simulink library "tqd"  (R2021b)
settings: Solver=VariableStepAuto  StartTime=0.0  StopTime=10.0  RelTol=1e-3
undefined symbols (not defined in the file or in its folder): ATQD_AccelLimitInRange_X_rpm, ATQD_AccelLimitInRange_Y_Nm, ATQD_AccelLimitOvrKi_X_Nm, ATQD_AccelLimitOvrKp_X_Nm, ATQD_BOSMapD_X_rpm, ATQD_BOSMapD_Y_pct, ATQD_BOSMapR_X_rpm, ATQD_BOSMapR_Y_pct, ATQD_HVBCurrSmooth_X_A, ATQD_LHMTqMapDLC_X_rpm, ATQD_LHMTqMapDLC_Y_pct, ATQD_LHMTqMapRLC_X_rpm, ATQD_LHMTqMapRLC_Y_pct, ATQD_NormalMapDLC_X_rpm, ATQD_NormalMapDLC_Y_pct, ATQD_NormalTqDecSR_X_rpm, ATQD_NormalTqDecSR_Y_Nm, ATQD_NormalTqIncSR_X_rpm, ATQD_NormalTqIncSR_Y_Nm, ATQD_OPDMapRLC_X_rpm, ATQD_OPDMapRLC_Y_pct, ATQD_RollRegTorReq_X_rpm, ATQD_RollRegTorReq_Y_enum, ATQD_VehSpdLimitInRange_X_rpm, ATQD_VehSpdLimitInRange_Y_Nm, ATQD_VehSpdLimitOvrKi_X_Nm, ATQD_VehSpdLimitOvrKp_X_Nm, EIGHT_INT, ENUM_BRAKEPEDAL_PRESSED, ENUM_BRAKEPEDAL_RELEASED, ENUM_COMBOKEY_DOWN, ENUM_COMBOKEY_M1, ENUM_COMBOKEY_M2, ENUM_COMBOKEY_NONE, ENUM_COMBOKEY_RKNEE, ENUM_COMBOKEY_STOPLV, ENUM_COMBOKEY_UP, ENUM_CP2VKNEEREQ_REQUEST, ENUM_CP2VNLVREQ_LEVEL1, ENUM_CP2VNLVREQ_LEVEL2, ENUM_CP2VNLVREQ_LOWER, ENUM_CP2VNLVREQ_STOPLV, ENUM_CP2VNLVREQ_UPPER, ENUM_CREEPIND_DISABLE, ENUM_CREEPIND_READY, ENUM_CREEPIND_RUNNING, ENUM_CREEPIND_WARNING, ENUM_DRIVELINERELEASE_RELEASE, ENUM_EBSTORQUERWQ_LIMIT, ENUM_EBSTORQUERWQ_TORQUE, ENUM_ECPVCUDRM_CONFORT, ENUM_ECPVCUDRM_ECO, ENUM_ECPVCUDRM_NORMAL, ENUM_ECPVCUDRM_NOTAVAILABLE, ENUM_EMTqModeDrvBrk_Accel, ENUM_EMTqModeDrvBrk_Brake, ENUM_EMTqModeDrvBrk_Coast, ENUM_ETC2ACTDRIVEDIR_BACKWARD, ENUM_ETC2ACTDRIVEDIR_FORWARD, ENUM_ETC2ACTDRIVEDIR_STILL ... (+341)
libraries: simulink x109, hcu_lib x67
(part 9 of 13)

== system tqd/TQD/Input_Convert/Input Signal Convert/Big Mike Combo V2 /Combo Key Detection/Function3 ==
  note: Manufacture Mode:
      | 11 = VINP_SWC2RRightSta_flg
      | 12 = VINP_SWC2RLeftSta_flg
      | 11 = VINP_SWC2RRightSta_flg
      | 12 = VINP_SWC2RLeftSta_flg
      | 11 = VINP_SWC2RRightSta_flg
      | 12 = VINP_SWC2RLeftSta_flg
      | 7 = VINP_SWC2LScrollPressSta_flg
      | 8 = VINP_SWC2LADASSta_flg
  task_time_s : Inport
  VTQD_ComboKeyEn_flg : Inport  Port=2
  VTQD_ComboKeyReset_flg : Inport  Port=3
  VTQD_ComboKey_enum : Inport  Port=4
  VTQD_ComboKeyEnter_flg : Inport  Port=5
  VTQD_ComboKeyOff_flg : Inport  Port=6
  AND : Logic  Inputs=9  AllPortsSameDT=off  OutDataTypeStr=boolean
  AND1 : Logic  AllPortsSameDT=off  OutDataTypeStr=boolean
  Constant : Constant  Value=ENUM_COMBOKEY_NONE
  Constant1 : Constant  Value=ENUM_COMBOKEY_NONE
  Constant2 : Constant  Value=FALSE
  Constant3 : Constant  Value=KTQD_ComboKeyDelay_s
  Delay : Delay  DelayLength=1  InitialCondition=uint8(0)
      settings: AttributesFormatString=%<InitialCondition>
  Delay1 : Delay  DelayLength=1  InitialCondition=uint8(0)
      settings: AttributesFormatString=%<InitialCondition>
  DelayEnable : hcu_lib/Basic_Blocks/DelayEnable
  Equal : RelationalOperator  Operator=~=  OutDataTypeStr=boolean  RndMeth=Simplest
  Key1 : Subsystem
      settings: RTWSystemCode=Nonreusable function
  Key2 : Subsystem
      settings: RTWSystemCode=Nonreusable function
  Key3 : Subsystem
      settings: RTWSystemCode=Nonreusable function
  Key4 : Subsystem
      settings: RTWSystemCode=Nonreusable function
  Key5 : Subsystem
      settings: RTWSystemCode=Nonreusable function
  Key6 : Subsystem
      settings: RTWSystemCode=Nonreusable function
  Key7 : Subsystem
      settings: RTWSystemCode=Nonreusable function
  Key8 : Subsystem
      settings: RTWSystemCode=Nonreusable function
  NOT : Logic  Operator=NOT  AllPortsSameDT=off  OutDataTypeStr=boolean
  Switch : Switch  Criteria=u2 ~= 0
      settings: AttributesFormatString=%<Criteria>
  Switch1 : Switch  Criteria=u2 ~= 0
      settings: AttributesFormatString=%<Criteria>
  Switch2 : Switch  Criteria=u2 ~= 0
      settings: AttributesFormatString=%<Criteria>
  VTQD_Function3Off_flg : Outport
  wires:
  [VTQD_Function3Off_flg] -> VTQD_Function3Off_flg/1
  Switch/1 -> [VTQD_Function3CMD_enum]  "VTQD_Function3CMD_enum"
  [task_time_s] -> DelayEnable/3
  Constant/1 -> Switch/3
  DelayEnable/1 -> Switch/2
  [VTQD_ComboKeyEn_flg] -> DelayEnable/1
  Constant3/1 -> DelayEnable/2
  [VTQD_ComboKey_enum] -> Switch/1
  [VTQD_Function3CMD_enum] -> Key1/1(VTQD_ComboKeyCMD_enum)
  [VTQD_ComboKeyEn_flg] -> Key1/2(VTQD_ComboKeyEn_flg)
  [VTQD_ComboKeyReset_flg] -> Key1/3(VTQD_ComboKeyReset_flg)
  [VTQD_Function3CMD_enum] -> Key2/1(VTQD_ComboKeyCMD_enum)
  [VTQD_ComboKeyEn_flg] -> Key2/2(VTQD_ComboKeyEn_flg)
  [VTQD_ComboKeyReset_flg] -> Key2/3(VTQD_ComboKeyReset_flg)
  [VTQD_ComboKey1_enum] -> Key2/4(VTQD_ComboKey1_enum)
  Key1/1(VTQD_ComboKey1_enum) -> [VTQD_ComboKey1_enum]
  Key1/2(VTQD_Key1Pass_flg) -> [VTQD_Key1Pass_flg]
  [VTQD_Function3CMD_enum] -> Key3/1(VTQD_ComboKeyCMD_enum)
  [VTQD_ComboKeyEn_flg] -> Key3/2(VTQD_ComboKeyEn_flg)
  [VTQD_ComboKeyReset_flg] -> Key3/3(VTQD_ComboKeyReset_flg)
  [VTQD_ComboKey2_enum] -> Key3/4(VTQD_ComboKey2_enum)
  [VTQD_Function3CMD_enum] -> Key4/1(VTQD_ComboKeyCMD_enum)
  [VTQD_ComboKeyEn_flg] -> Key4/2(VTQD_ComboKeyEn_flg)
  [VTQD_ComboKeyReset_flg] -> Key4/3(VTQD_ComboKeyReset_flg)
  Key2/1(VTQD_ComboKey2_enum) -> [VTQD_ComboKey2_enum]
  Key2/2(VTQD_Key2Pass_flg) -> [VTQD_Key2Pass_flg]
  [VTQD_ComboKey3_enum] -> Key4/4(VTQD_ComboKey3_enum)
  Key3/1(VTQD_ComboKey3_enum) -> [VTQD_ComboKey3_enum]
  Key3/2(VTQD_Key3Pass_flg) -> [VTQD_Key3Pass_flg]
  Key4/1(VTQD_ComboKey4_enum) -> [VTQD_ComboKey4_enum]
  Key4/2(VTQD_Key4Pass_flg) -> [VTQD_Key4Pass_flg]
  [VTQD_ComboKeyReset_flg] -> Key5/3(VTQD_ComboKeyReset_flg)
  [VTQD_ComboKeyEn_flg] -> Key5/2(VTQD_ComboKeyEn_flg)
  [VTQD_Function3CMD_enum] -> Key5/1(VTQD_ComboKeyCMD_enum)
  [VTQD_ComboKey4_enum] -> Key5/4(VTQD_ComboKey4_enum)
  Key5/2(VTQD_Key5Pass_flg) -> [VTQD_Key5Pass_flg]
  Key5/1(VTQD_ComboKey5_enum) -> [VTQD_ComboKey5_enum]
  Key7/2(VTQD_Key7Pass_flg) -> [VTQD_Key7Pass_flg]
  Key8/1(VTQD_ComboKey8_enum) -> [VTQD_ComboKey8_enum]
  Key8/2(VTQD_Key8Pass_flg) -> [VTQD_Key8Pass_flg]
  [VTQD_Function3CMD_enum] -> Key6/1(VTQD_ComboKeyCMD_enum)
  [VTQD_ComboKeyEn_flg] -> Key6/2(VTQD_ComboKeyEn_flg)
  [VTQD_ComboKeyReset_flg] -> Key6/3(VTQD_ComboKeyReset_flg)
  [VTQD_ComboKey5_enum] -> Key6/4(VTQD_ComboKey5_enum)
  [VTQD_Function3CMD_enum] -> Key7/1(VTQD_ComboKeyCMD_enum)
  [VTQD_ComboKeyEn_flg] -> Key7/2(VTQD_ComboKeyEn_flg)
  [VTQD_ComboKeyReset_flg] -> Key7/3(VTQD_ComboKeyReset_flg)
  [VTQD_ComboKey6_enum] -> Key7/4(VTQD_ComboKey6_enum)
  [VTQD_Function3CMD_enum] -> Key8/1(VTQD_ComboKeyCMD_enum)
  [VTQD_ComboKeyEn_flg] -> Key8/2(VTQD_ComboKeyEn_flg)
  [VTQD_ComboKeyReset_flg] -> Key8/3(VTQD_ComboKeyReset_flg)
  [VTQD_ComboKey7_enum] -> Key8/4(VTQD_ComboKey7_enum)
  Constant1/1 -> Equal/2
  Equal/1 -> AND/1
  [VTQD_Key1Pass_flg] -> AND/2
  [VTQD_Key8Pass_flg] -> AND/9
  [VTQD_Key7Pass_flg] -> AND/8
  [VTQD_Key6Pass_flg] -> AND/7
  [VTQD_Key5Pass_flg] -> AND/6
  [VTQD_Key4Pass_flg] -> AND/5
  [VTQD_Key3Pass_flg] -> AND/4
  [VTQD_Key2Pass_flg] -> AND/3
  AND/1 -> Switch1/1  "VTQD_Function3OffPass_flg"
  Switch1/1 -> Switch2/3
  [VTQD_ComboKeyOff_flg] -> Switch2/2
  Constant2/1 -> Switch2/1
  Switch2/1 -> Delay/1, [VTQD_Function3Off_flg]  "VTQD_Function3Off_flg"
  Delay/1 -> Switch1/3
  task_time_s/1 -> [task_time_s]
  VTQD_ComboKeyEn_flg/1 -> [VTQD_ComboKeyEn_flg]
  VTQD_ComboKeyReset_flg/1 -> [VTQD_ComboKeyReset_flg]
  VTQD_ComboKey_enum/1 -> [VTQD_ComboKey_enum]
  VTQD_ComboKeyEnter_flg/1 -> [VTQD_ComboKeyEnter_flg]
  VTQD_ComboKeyOff_flg/1 -> [VTQD_ComboKeyOff_flg]
  Key6/1(VTQD_ComboKey6_enum) -> [VTQD_ComboKey6_enum]
  Key6/2(VTQD_Key6Pass_flg) -> [VTQD_Key6Pass_flg]
  Key7/1(VTQD_ComboKey7_enum) -> [VTQD_ComboKey7_enum]
  [VTQD_ComboKey8_enum] -> Equal/1
  NOT/1 -> AND1/2
  Delay1/1 -> NOT/1
  [VTQD_ComboKeyEnter_flg] -> AND1/1
  AND1/1 -> Switch1/2
  [VTQD_Function3Off_flg] -> Delay1/1

== system tqd/TQD/Input_Convert/Input Signal Convert/Big Mike Combo V2 /Combo Key Detection/Function4  ==
  note: Exhibition Mode:
      | 7 = VINP_SWC2LScrollPressSta_flg
      | 7 = VINP_SWC2LScrollPressSta_flg
      | 8 = VINP_SWC2LADASSta_flg
      | 8 = VINP_SWC2LADASSta_flg
      | 8 = VINP_SWC2LADASSta_flg
      | 7 = VINP_SWC2LScrollPressSta_flg
      | 8 = VINP_SWC2LADASSta_flg
      | 7 = VINP_SWC2LScrollPressSta_flg
  task_time_s : Inport
  VTQD_ComboKeyEn_flg : Inport  Port=2
  VTQD_ComboKeyReset_flg : Inport  Port=3
  VTQD_ComboKey_enum : Inport  Port=4
  VTQD_ComboKeyEnter_flg : Inport  Port=5
  VTQD_ComboKeyOff_flg : Inport  Port=6
  AND : Logic  Inputs=9  AllPortsSameDT=off  OutDataTypeStr=boolean
  AND1 : Logic  AllPortsSameDT=off  OutDataTypeStr=boolean
  Constant : Constant  Value=ENUM_COMBOKEY_NONE
  Constant1 : Constant  Value=ENUM_COMBOKEY_NONE
  Constant2 : Constant  Value=FALSE
  Constant3 : Constant  Value=KTQD_ComboKeyDelay_s
  Delay : Delay  DelayLength=1  InitialCondition=boolean(0)
      settings: AttributesFormatString=%<InitialCondition>
  Delay1 : Delay  DelayLength=1  InitialCondition=boolean(0)
      settings: AttributesFormatString=%<InitialCondition>
  DelayEnable : hcu_lib/Basic_Blocks/DelayEnable
  Equal : RelationalOperator  Operator=~=  OutDataTypeStr=boolean  RndMeth=Simplest
  Key1 : Subsystem
      settings: RTWSystemCode=Nonreusable function
  Key2 : Subsystem
      settings: RTWSystemCode=Nonreusable function
  Key3 : Subsystem
      settings: RTWSystemCode=Nonreusable function
  Key4 : Subsystem
      settings: RTWSystemCode=Nonreusable function
  Key5 : Subsystem
      settings: RTWSystemCode=Nonreusable function
  Key6 : Subsystem
      settings: RTWSystemCode=Nonreusable function
  Key7 : Subsystem
      settings: RTWSystemCode=Nonreusable function
  Key8 : Subsystem
      settings: RTWSystemCode=Nonreusable function
  NOT : Logic  Operator=NOT  AllPortsSameDT=off  OutDataTypeStr=boolean
  Switch : Switch  Criteria=u2 ~= 0
      settings: AttributesFormatString=%<Criteria>
  Switch1 : Switch  Criteria=u2 ~= 0
      settings: AttributesFormatString=%<Criteria>
  Switch2 : Switch  Criteria=u2 ~= 0
      settings: AttributesFormatString=%<Criteria>
  VTQD_Function4Off_flg : Outport
  wires:
  [VTQD_ComboKey8_enum] -> Equal/1
  Key7/1(VTQD_ComboKey7_enum) -> [VTQD_ComboKey7_enum]
  Key6/2(VTQD_Key6Pass_flg) -> [VTQD_Key6Pass_flg]
  Key6/1(VTQD_ComboKey6_enum) -> [VTQD_ComboKey6_enum]
  VTQD_ComboKeyOff_flg/1 -> [VTQD_ComboKeyOff_flg]
  VTQD_ComboKeyEnter_flg/1 -> [VTQD_ComboKeyEnter_flg]
  VTQD_ComboKey_enum/1 -> [VTQD_ComboKey_enum]
  VTQD_ComboKeyReset_flg/1 -> [VTQD_ComboKeyReset_flg]
  VTQD_ComboKeyEn_flg/1 -> [VTQD_ComboKeyEn_flg]
  task_time_s/1 -> [task_time_s]
  Delay/1 -> Switch1/3
  Switch2/1 -> [VTQD_Function4Off_flg], Delay/1  "VTQD_Function4Off_flg"
  Constant2/1 -> Switch2/1
  [VTQD_ComboKeyOff_flg] -> Switch2/2
  Switch1/1 -> Switch2/3
  AND/1 -> Switch1/1  "VTQD_Function4OffPass_flg"
  [VTQD_Key2Pass_flg] -> AND/3
  [VTQD_Key3Pass_flg] -> AND/4
  [VTQD_Key4Pass_flg] -> AND/5
  [VTQD_Key5Pass_flg] -> AND/6
  [VTQD_Key6Pass_flg] -> AND/7
  [VTQD_Key7Pass_flg] -> AND/8
  [VTQD_Key8Pass_flg] -> AND/9
  [VTQD_Key1Pass_flg] -> AND/2
  Equal/1 -> AND/1
  Constant1/1 -> Equal/2
  [VTQD_ComboKey7_enum] -> Key8/4(VTQD_ComboKey7_enum)
  [VTQD_ComboKeyReset_flg] -> Key8/3(VTQD_ComboKeyReset_flg)
  [VTQD_ComboKeyEn_flg] -> Key8/2(VTQD_ComboKeyEn_flg)
  [VTQD_Function4CMD_enum] -> Key8/1(VTQD_ComboKeyCMD_enum)
  [VTQD_ComboKey6_enum] -> Key7/4(VTQD_ComboKey6_enum)
  [VTQD_ComboKeyReset_flg] -> Key7/3(VTQD_ComboKeyReset_flg)
  [VTQD_ComboKeyEn_flg] -> Key7/2(VTQD_ComboKeyEn_flg)
  [VTQD_Function4CMD_enum] -> Key7/1(VTQD_ComboKeyCMD_enum)
  [VTQD_ComboKey5_enum] -> Key6/4(VTQD_ComboKey5_enum)
  [VTQD_ComboKeyReset_flg] -> Key6/3(VTQD_ComboKeyReset_flg)
  [VTQD_ComboKeyEn_flg] -> Key6/2(VTQD_ComboKeyEn_flg)
  [VTQD_Function4CMD_enum] -> Key6/1(VTQD_ComboKeyCMD_enum)
  Key8/2(VTQD_Key8Pass_flg) -> [VTQD_Key8Pass_flg]
  Key8/1(VTQD_ComboKey8_enum) -> [VTQD_ComboKey8_enum]
  Key7/2(VTQD_Key7Pass_flg) -> [VTQD_Key7Pass_flg]
  Key5/1(VTQD_ComboKey5_enum) -> [VTQD_ComboKey5_enum]
  Key5/2(VTQD_Key5Pass_flg) -> [VTQD_Key5Pass_flg]
  [VTQD_ComboKey4_enum] -> Key5/4(VTQD_ComboKey4_enum)
  [VTQD_Function4CMD_enum] -> Key5/1(VTQD_ComboKeyCMD_enum)
  [VTQD_ComboKeyEn_flg] -> Key5/2(VTQD_ComboKeyEn_flg)
  [VTQD_ComboKeyReset_flg] -> Key5/3(VTQD_ComboKeyReset_flg)
  Key4/2(VTQD_Key4Pass_flg) -> [VTQD_Key4Pass_flg]
  Key4/1(VTQD_ComboKey4_enum) -> [VTQD_ComboKey4_enum]
  Key3/2(VTQD_Key3Pass_flg) -> [VTQD_Key3Pass_flg]
  Key3/1(VTQD_ComboKey3_enum) -> [VTQD_ComboKey3_enum]
  [VTQD_ComboKey3_enum] -> Key4/4(VTQD_ComboKey3_enum)
  Key2/2(VTQD_Key2Pass_flg) -> [VTQD_Key2Pass_flg]
  Key2/1(VTQD_ComboKey2_enum) -> [VTQD_ComboKey2_enum]
  [VTQD_ComboKeyReset_flg] -> Key4/3(VTQD_ComboKeyReset_flg)
  [VTQD_ComboKeyEn_flg] -> Key4/2(VTQD_ComboKeyEn_flg)
  [VTQD_Function4CMD_enum] -> Key4/1(VTQD_ComboKeyCMD_enum)
  [VTQD_ComboKey2_enum] -> Key3/4(VTQD_ComboKey2_enum)
  [VTQD_ComboKeyReset_flg] -> Key3/3(VTQD_ComboKeyReset_flg)
  [VTQD_ComboKeyEn_flg] -> Key3/2(VTQD_ComboKeyEn_flg)
  [VTQD_Function4CMD_enum] -> Key3/1(VTQD_ComboKeyCMD_enum)
  Key1/2(VTQD_Key1Pass_flg) -> [VTQD_Key1Pass_flg]
  Key1/1(VTQD_ComboKey1_enum) -> [VTQD_ComboKey1_enum]
  [VTQD_ComboKey1_enum] -> Key2/4(VTQD_ComboKey1_enum)
  [VTQD_ComboKeyReset_flg] -> Key2/3(VTQD_ComboKeyReset_flg)
  [VTQD_ComboKeyEn_flg] -> Key2/2(VTQD_ComboKeyEn_flg)
  [VTQD_Function4CMD_enum] -> Key2/1(VTQD_ComboKeyCMD_enum)
  [VTQD_ComboKeyReset_flg] -> Key1/3(VTQD_ComboKeyReset_flg)
  [VTQD_ComboKeyEn_flg] -> Key1/2(VTQD_ComboKeyEn_flg)
  [VTQD_Function4CMD_enum] -> Key1/1(VTQD_ComboKeyCMD_enum)
  [VTQD_ComboKey_enum] -> Switch/1
  Constant3/1 -> DelayEnable/2
  [VTQD_ComboKeyEn_flg] -> DelayEnable/1
  DelayEnable/1 -> Switch/2
  Constant/1 -> Switch/3
  [task_time_s] -> DelayEnable/3
  Switch/1 -> [VTQD_Function4CMD_enum]  "VTQD_Function4CMD_enum"
  [VTQD_Function4Off_flg] -> VTQD_Function4Off_flg/1
  NOT/1 -> AND1/2
  Delay1/1 -> NOT/1
  [VTQD_Function4Off_flg] -> Delay1/1
  [VTQD_ComboKeyEnter_flg] -> AND1/1
  AND1/1 -> Switch1/2

== system tqd/TQD/Input_Convert/Input Signal Convert/Big Mike Combo V2 /Combo Key Detection/Function5 ==
  note: Exhibition Mode:
      | 1 = VINP_SWC2RegenDown_flg
      | 2 = VINP_SWC2RegenUp_flg
      | 3 = VINP_SWC2LScrollUpSta_flg
      | 4 = VINP_SWC2LScrollDownSta_flg
      | 5 = VINP_SWC2RScrollUpSta_flg
      | 6 = VINP_SWC2RScrollDownSta_flg
      | 7 = VINP_SWC2LScrollPressSta_flg
      | 8 = VINP_SWC2LADASSta_flg
  task_time_s : Inport
  VTQD_ComboKeyEn_flg : Inport  Port=2
  VTQD_ComboKeyReset_flg : Inport  Port=3
  VTQD_ComboKey_enum : Inport  Port=4
  VTQD_ComboKeyEnter_flg : Inport  Port=5
  VTQD_ComboKeyOff_flg : Inport  Port=6
  AND : Logic  Inputs=9  AllPortsSameDT=off  OutDataTypeStr=boolean
  AND1 : Logic  AllPortsSameDT=off  OutDataTypeStr=boolean
  Constant : Constant  Value=ENUM_COMBOKEY_NONE
  Constant1 : Constant  Value=ENUM_COMBOKEY_NONE
  Constant2 : Constant  Value=FALSE
  Constant3 : Constant  Value=KTQD_ComboKeyDelay_s
  Delay : Delay  DelayLength=1  InitialCondition=uint8(0)
      settings: AttributesFormatString=%<InitialCondition>
  Delay1 : Delay  DelayLength=1  InitialCondition=boolean(0)
      settings: AttributesFormatString=%<InitialCondition>
  DelayEnable : hcu_lib/Basic_Blocks/DelayEnable
  Equal : RelationalOperator  Operator=~=  OutDataTypeStr=boolean  RndMeth=Simplest
  Key1 : Subsystem
      settings: RTWSystemCode=Nonreusable function
  Key2 : Subsystem
      settings: RTWSystemCode=Nonreusable function
  Key3 : Subsystem
      settings: RTWSystemCode=Nonreusable function
  Key4 : Subsystem
      settings: RTWSystemCode=Nonreusable function
  Key5 : Subsystem
      settings: RTWSystemCode=Nonreusable function
  Key6 : Subsystem
      settings: RTWSystemCode=Nonreusable function
  Key7 : Subsystem
      settings: RTWSystemCode=Nonreusable function
  Key8 : Subsystem
      settings: RTWSystemCode=Nonreusable function
  NOT : Logic  Operator=NOT  AllPortsSameDT=off  OutDataTypeStr=boolean
  Switch : Switch  Criteria=u2 ~= 0
      settings: AttributesFormatString=%<Criteria>
  Switch1 : Switch  Criteria=u2 ~= 0
      settings: AttributesFormatString=%<Criteria>
  Switch2 : Switch  Criteria=u2 ~= 0
      settings: AttributesFormatString=%<Criteria>
  VTQD_Function5Off_flg : Outport
  wires:
  [VTQD_Function5Off_flg] -> VTQD_Function5Off_flg/1
  Switch/1 -> [VTQD_Function5CMD_enum]  "VTQD_Function5CMD_enum"
  [task_time_s] -> DelayEnable/3
  Constant/1 -> Switch/3
  DelayEnable/1 -> Switch/2
  [VTQD_ComboKeyEn_flg] -> DelayEnable/1
  Constant3/1 -> DelayEnable/2
  [VTQD_ComboKey_enum] -> Switch/1
  [VTQD_Function5CMD_enum] -> Key1/1(VTQD_ComboKeyCMD_enum)
  [VTQD_ComboKeyEn_flg] -> Key1/2(VTQD_ComboKeyEn_flg)
  [VTQD_ComboKeyReset_flg] -> Key1/3(VTQD_ComboKeyReset_flg)
  [VTQD_Function5CMD_enum] -> Key2/1(VTQD_ComboKeyCMD_enum)
  [VTQD_ComboKeyEn_flg] -> Key2/2(VTQD_ComboKeyEn_flg)
  [VTQD_ComboKeyReset_flg] -> Key2/3(VTQD_ComboKeyReset_flg)
  [VTQD_ComboKey1_enum] -> Key2/4(VTQD_ComboKey1_enum)
  Key1/1(VTQD_ComboKey1_enum) -> [VTQD_ComboKey1_enum]
  Key1/2(VTQD_Key1Pass_flg) -> [VTQD_Key1Pass_flg]
  [VTQD_Function5CMD_enum] -> Key3/1(VTQD_ComboKeyCMD_enum)
  [VTQD_ComboKeyEn_flg] -> Key3/2(VTQD_ComboKeyEn_flg)
  [VTQD_ComboKeyReset_flg] -> Key3/3(VTQD_ComboKeyReset_flg)
  [VTQD_ComboKey2_enum] -> Key3/4(VTQD_ComboKey2_enum)
  [VTQD_Function5CMD_enum] -> Key4/1(VTQD_ComboKeyCMD_enum)
  [VTQD_ComboKeyEn_flg] -> Key4/2(VTQD_ComboKeyEn_flg)
  [VTQD_ComboKeyReset_flg] -> Key4/3(VTQD_ComboKeyReset_flg)
  Key2/1(VTQD_ComboKey2_enum) -> [VTQD_ComboKey2_enum]
  Key2/2(VTQD_Key2Pass_flg) -> [VTQD_Key2Pass_flg]
  [VTQD_ComboKey3_enum] -> Key4/4(VTQD_ComboKey3_enum)
  Key3/1(VTQD_ComboKey3_enum) -> [VTQD_ComboKey3_enum]
  Key3/2(VTQD_Key3Pass_flg) -> [VTQD_Key3Pass_flg]
  Key4/1(VTQD_ComboKey4_enum) -> [VTQD_ComboKey4_enum]
  Key4/2(VTQD_Key4Pass_flg) -> [VTQD_Key4Pass_flg]
  [VTQD_ComboKeyReset_flg] -> Key5/3(VTQD_ComboKeyReset_flg)
  [VTQD_ComboKeyEn_flg] -> Key5/2(VTQD_ComboKeyEn_flg)
  [VTQD_Function5CMD_enum] -> Key5/1(VTQD_ComboKeyCMD_enum)
  [VTQD_ComboKey4_enum] -> Key5/4(VTQD_ComboKey4_enum)
  Key5/2(VTQD_Key5Pass_flg) -> [VTQD_Key5Pass_flg]
  Key5/1(VTQD_ComboKey5_enum) -> [VTQD_ComboKey5_enum]
  Key7/2(VTQD_Key7Pass_flg) -> [VTQD_Key7Pass_flg]
  Key8/1(VTQD_ComboKey8_enum) -> [VTQD_ComboKey8_enum]
  Key8/2(VTQD_Key8Pass_flg) -> [VTQD_Key8Pass_flg]
  [VTQD_Function5CMD_enum] -> Key6/1(VTQD_ComboKeyCMD_enum)
  [VTQD_ComboKeyEn_flg] -> Key6/2(VTQD_ComboKeyEn_flg)
  [VTQD_ComboKeyReset_flg] -> Key6/3(VTQD_ComboKeyReset_flg)
  [VTQD_ComboKey5_enum] -> Key6/4(VTQD_ComboKey5_enum)
  [VTQD_Function5CMD_enum] -> Key7/1(VTQD_ComboKeyCMD_enum)
  [VTQD_ComboKeyEn_flg] -> Key7/2(VTQD_ComboKeyEn_flg)
  [VTQD_ComboKeyReset_flg] -> Key7/3(VTQD_ComboKeyReset_flg)
  [VTQD_ComboKey6_enum] -> Key7/4(VTQD_ComboKey6_enum)
  [VTQD_Function5CMD_enum] -> Key8/1(VTQD_ComboKeyCMD_enum)
  [VTQD_ComboKeyEn_flg] -> Key8/2(VTQD_ComboKeyEn_flg)
  [VTQD_ComboKeyReset_flg] -> Key8/3(VTQD_ComboKeyReset_flg)
  [VTQD_ComboKey7_enum] -> Key8/4(VTQD_ComboKey7_enum)
  Constant1/1 -> Equal/2
  Equal/1 -> AND/1
  [VTQD_Key1Pass_flg] -> AND/2
  [VTQD_Key8Pass_flg] -> AND/9
  [VTQD_Key7Pass_flg] -> AND/8
  [VTQD_Key6Pass_flg] -> AND/7
  [VTQD_Key5Pass_flg] -> AND/6
  [VTQD_Key4Pass_flg] -> AND/5
  [VTQD_Key3Pass_flg] -> AND/4
  [VTQD_Key2Pass_flg] -> AND/3
  AND/1 -> Switch1/1  "VTQD_Function5OffPass_flg"
  Switch1/1 -> Switch2/3
  [VTQD_ComboKeyOff_flg] -> Switch2/2
  Constant2/1 -> Switch2/1
  Switch2/1 -> [VTQD_Function5Off_flg], Delay/1  "VTQD_Function5Off_flg"
  Delay/1 -> Switch1/3
  task_time_s/1 -> [task_time_s]
  VTQD_ComboKeyEn_flg/1 -> [VTQD_ComboKeyEn_flg]
  VTQD_ComboKeyReset_flg/1 -> [VTQD_ComboKeyReset_flg]
  VTQD_ComboKey_enum/1 -> [VTQD_ComboKey_enum]
  VTQD_ComboKeyEnter_flg/1 -> [VTQD_ComboKeyEnter_flg]
  VTQD_ComboKeyOff_flg/1 -> [VTQD_ComboKeyOff_flg]
  Key6/1(VTQD_ComboKey6_enum) -> [VTQD_ComboKey6_enum]
  Key6/2(VTQD_Key6Pass_flg) -> [VTQD_Key6Pass_flg]
  Key7/1(VTQD_ComboKey7_enum) -> [VTQD_ComboKey7_enum]
  [VTQD_ComboKey8_enum] -> Equal/1
  NOT/1 -> AND1/2
  Delay1/1 -> NOT/1
  [VTQD_ComboKeyEnter_flg] -> AND1/1
  [VTQD_Function5Off_flg] -> Delay1/1
  AND1/1 -> Switch1/2

== system tqd/TQD/Input_Convert/Input Signal Convert/Big Mike Combo V2 /Signal Status Detection/DownShort ==
  Action Port : ActionPort
  Constant : Constant  Value=ENUM_COMBOKEY_DOWN  OutDataTypeStr=uint8
  DownShort : Outport
  wires:
  Constant/1 -> DownShort/1

== system tqd/TQD/Input_Convert/Input Signal Convert/Big Mike Combo V2 /Signal Status Detection/M1Short ==
  Action Port : ActionPort
  Constant : Constant  Value=ENUM_COMBOKEY_M1  OutDataTypeStr=uint8
  M1Short : Outport
  wires:
  Constant/1 -> M1Short/1

== system tqd/TQD/Input_Convert/Input Signal Convert/Big Mike Combo V2 /Signal Status Detection/M2Short ==
  Action Port : ActionPort
  Constant : Constant  Value=ENUM_COMBOKEY_M2  OutDataTypeStr=uint8
  M2Short : Outport
  wires:
  Constant/1 -> M2Short/1

== system tqd/TQD/Input_Convert/Input Signal Convert/Big Mike Combo V2 /Signal Status Detection/None ==
  Action Port : ActionPort
  Constant : Constant  Value=ENUM_COMBOKEY_NONE  OutDataTypeStr=uint8
  None : Outport
  wires:
  Constant/1 -> None/1

== system tqd/TQD/Input_Convert/Input Signal Convert/Big Mike Combo V2 /Signal Status Detection/RKneeShort ==
  Action Port : ActionPort
  Constant : Constant  Value=ENUM_COMBOKEY_RKNEE  OutDataTypeStr=uint8
  RKneeShort : Outport
  wires:
  Constant/1 -> RKneeShort/1

== system tqd/TQD/Input_Convert/Input Signal Convert/Big Mike Combo V2 /Signal Status Detection/StopLVShort ==
  Action Port : ActionPort
  Constant : Constant  Value=ENUM_COMBOKEY_STOPLV  OutDataTypeStr=uint8
  STOPLV : Outport
  wires:
  Constant/1 -> STOPLV/1

== system tqd/TQD/Input_Convert/Input Signal Convert/Big Mike Combo V2 /Signal Status Detection/Street Fight Switch Off ==
  task_time_s : Inport
  VTQD_SWCCANCELStaShort_flg : Inport  Port=2
  VTQD_ComboKeyPreEn_flg : Inport  Port=3
  SWCCANCELStaLong_flg : Inport  Port=4
  VTQD_FunctionOffSta_enum : Inport  Port=5
  AND : Logic  AllPortsSameDT=off  OutDataTypeStr=boolean
  AND2 : Logic  AllPortsSameDT=off  OutDataTypeStr=boolean
  Add : Sum
  Constant1 : Constant  Value=ZERO_INT
  Constant11 : Constant  Value=ONE_INT
  Constant2 : Constant  Value=ONE_INT
  Constant3 : Constant  Value=KTQD_CANCELUpCount_cnt
  Constant4 : Constant  Value=ZERO_INT
  Constant5 : Constant  Value=ZERO_INT
  Constant6 : Constant  Value=KTQD_ComboKeyOff_flg_ovrdflg
  Constant7 : Constant  Value=KTQD_CANCELCountDetTime_s
  Constant8 : Constant  Value=KTQD_ComboKeyOff_flg_ovrdval
  Delay : Delay  DelayLength=1  InitialCondition=uint8(0)
      settings: AttributesFormatString=%<InitialCondition>
  Delay1 : Delay  DelayLength=1  InitialCondition=boolean(0)
      settings: AttributesFormatString=%<InitialCondition>
  Delay2 : Delay  DelayLength=1  InitialCondition=boolean(0)
      settings: AttributesFormatString=%<InitialCondition>
  Delay3 : Delay  DelayLength=1  InitialCondition=uint8(0)
      settings: AttributesFormatString=%<InitialCondition>
  Equal : RelationalOperator  Operator===  OutDataTypeStr=boolean  RndMeth=Simplest
  Equal1 : RelationalOperator  Operator===  OutDataTypeStr=boolean  RndMeth=Simplest
  Equal2 : RelationalOperator  Operator=>  OutDataTypeStr=boolean  RndMeth=Simplest
  NOT : Logic  Operator=NOT  AllPortsSameDT=off  OutDataTypeStr=boolean
  NOT1 : Logic  Operator=NOT  AllPortsSameDT=off  OutDataTypeStr=boolean
  OR : Logic  Operator=OR  Inputs=3  AllPortsSameDT=off  OutDataTypeStr=boolean
  Relational Operator : RelationalOperator  OutDataTypeStr=boolean  RndMeth=Simplest
  SR_Latch : hcu_lib/Basic_Blocks/SR_Latch
  Switch : Switch  Criteria=u2 ~= 0
      settings: AttributesFormatString=%<Criteria>
  Switch1 : Switch  Criteria=u2 ~= 0
      settings: AttributesFormatString=%<Criteria>
  Switch2 : Switch  Criteria=u2 ~= 0
      settings: AttributesFormatString=%<Criteria>
  Timer : hcu_lib/Basic_Blocks/Timer
  VTQD_ComboKeyOff_flg : Outport
  wires:
  Constant1/1 -> Switch/3
  [VTQD_SWCCANCELStaShort_flg] -> Switch/2
  Constant11/1 -> Switch/1
  Switch/1 -> Add/1
  Add/1 -> Switch1/3
  Switch1/1 -> [VTQD_CANCELCount_cnt], Delay/1  "VTQD_CANCELCount_cnt"
  Delay/1 -> Add/2
  [VTQD_CANCELCount_cnt] -> Equal/1
  Constant2/1 -> Equal/2
  Equal/1 -> AND/1
  [VTQD_ComboKeyPreEn_flg] -> AND/2
  AND/1 -> SR_Latch/1
  SR_Latch/1 -> NOT/1, Timer/1
  NOT/1 -> Timer/2
  [task_time_s] -> Timer/3
  Constant7/1 -> Relational Operator/2, Timer/4
  Timer/1 -> Relational Operator/1  "VTQD_CANCELCountDetTime_s"
  Relational Operator/1 -> [VTQD_CANCELCountDetFinish_flg]  "VTQD_CANCELCountDetFinish_flg"
  [VTQD_CANCELCount_cnt] -> Equal1/1
  Constant3/1 -> Equal1/2
  [SWCCANCELStaLong_flg] -> AND2/2
  [VTQD_CANCELCountDetFinish_flg] -> Delay1/1
  Delay1/1 -> SR_Latch/2
  [VTQD_CANCELCountDetFinish_flg] -> Delay2/1
  Constant4/1 -> Switch1/1
  Equal1/1 -> AND2/1
  task_time_s/1 -> [task_time_s]
  VTQD_SWCCANCELStaShort_flg/1 -> [VTQD_SWCCANCELStaShort_flg]
  VTQD_ComboKeyPreEn_flg/1 -> [VTQD_ComboKeyPreEn_flg]
  SWCCANCELStaLong_flg/1 -> [SWCCANCELStaLong_flg]
  [VTQD_ComboKeyOff_flg] -> VTQD_ComboKeyOff_flg/1
  [VTQD_ComboKeyPreEn_flg] -> NOT1/1
  VTQD_FunctionOffSta_enum/1 -> [VTQD_FunctionOffSta_enum]
  Equal2/1 -> OR/1
  NOT1/1 -> OR/2
  Delay2/1 -> OR/3
  OR/1 -> [VTQD_CANCELCountReset_flg]  "VTQD_CANCELCountReset_flg"
  [VTQD_CANCELCountReset_flg] -> Switch1/2
  [VTQD_FunctionOffSta_enum] -> Delay3/1
  Delay3/1 -> Equal2/1
  Constant5/1 -> Equal2/2
  AND2/1 -> Switch2/3
  Constant6/1 -> Switch2/2
  Constant8/1 -> Switch2/1
  Switch2/1 -> [VTQD_ComboKeyOff_flg]  "VTQD_ComboKeyOff_flg"

== system tqd/TQD/Input_Convert/Input Signal Convert/Big Mike Combo V2 /Signal Status Detection/UpShort ==
  Action Port : ActionPort
  Constant : Constant  Value=ENUM_COMBOKEY_UP  OutDataTypeStr=uint8
  UpShort : Outport
  wires:
  Constant/1 -> UpShort/1

== system tqd/TQD/Input_Convert/Input Signal Convert/Big Mike Combo V2 /Combo Key Detection/Function1 Alcohol Lock/Key1 ==
  VTQD_ComboKeyCMD_enum : Inport
  VTQD_ComboKeyEn_flg : Inport  Port=2
  VTQD_ComboKeyReset_flg : Inport  Port=3
  AND : Logic  Inputs=3  AllPortsSameDT=off  OutDataTypeStr=boolean
  Constant1 : Constant  Value=KTQD_Function1Off1_enum
  Constant2 : Constant  Value=ENUM_COMBOKEY_NONE
  Constant4 : Constant  Value=ENUM_COMBOKEY_NONE
  Data Type Conversion : DataTypeConversion  OutDataTypeStr=uint8
  Delay : Delay  DelayLength=1  InitialCondition=uint8(0)
      settings: AttributesFormatString=%<InitialCondition>
  Delay1 : Delay  DelayLength=1  InitialCondition=uint8(0)
      settings: AttributesFormatString=%<InitialCondition>
  Detect Change : simulink/Logic and Bit Operations/Detect Change  vinit=boolean(0)  OutDataTypeStr=boolean
  Detect Increase : simulink/Logic and Bit Operations/Detect Increase  vinit=boolean(0)  OutDataTypeStr=boolean
  Equal : RelationalOperator  Operator===  OutDataTypeStr=boolean  RndMeth=Simplest
  Equal1 : RelationalOperator  Operator=~=  OutDataTypeStr=boolean  RndMeth=Simplest
  Equal2 : RelationalOperator  Operator===  OutDataTypeStr=boolean  RndMeth=Simplest
  If : If  NumInputs=2  IfExpression=u1 ~=0  ElseIfExpressions=u2 ~= 0
  Maintain : Subsystem  TreatAsAtomicUnit=on
  Merge : Merge  Inputs=3
  OR : Logic  Operator=OR  AllPortsSameDT=off  OutDataTypeStr=boolean
  Reset : Subsystem  TreatAsAtomicUnit=on
  Write : Subsystem  TreatAsAtomicUnit=on
  VTQD_ComboKey1_enum : Outport
  VTQD_Key1Pass_flg : Outport  Port=2
  wires:
  OR/1 -> [VTQD_ResetComboKey_flg]  "VTQD_ResetComboKey_flg"
  [VTQD_WriteComboCMD_flg] -> If/2
  [VTQD_ComboKeyCMD_enum] -> Equal1/1
  [VTQD_ComboKeyReset_flg] -> OR/2
  [VTQD_ComboKey1_enum] -> Delay/1
  Equal1/1 -> AND/2
  Constant2/1 -> Equal2/2
  Equal2/1 -> AND/3
  Reset/1(ResetToZero) -> Merge/1
  Merge/1 -> Data Type Conversion/1
  Delay/1 -> Equal2/1
  If/3 -> Maintain/Action
  Constant4/1 -> Equal1/2
  Maintain/1(KeepKey1) -> Merge/3
  Detect Change/1 -> AND/1
  [VTQD_ComboKeyEn_flg] -> Detect Increase/1
  [VTQD_ResetComboKey_flg] -> If/1
  [VTQD_ComboKeyCMD_enum] -> Detect Change/1
  [VTQD_ComboKeyCMD_enum] -> Write/1(Input)
  AND/1 -> [VTQD_WriteComboCMD_flg]  "VTQD_WriteComboCMD_flg"
  Detect Increase/1 -> OR/1
  If/1 -> Reset/Action
  Write/1(WriteCMD) -> Merge/2
  If/2 -> Write/Action
  [VTQD_ComboKey1_enum] -> Equal/1
  Constant1/1 -> Equal/2
  Equal/1 -> [VTQD_Function1Off1Pass_flg]  "VTQD_Function1Off1Pass_flg"
  VTQD_ComboKeyCMD_enum/1 -> [VTQD_ComboKeyCMD_enum]
  VTQD_ComboKeyReset_flg/1 -> [VTQD_ComboKeyReset_flg]
  VTQD_ComboKeyEn_flg/1 -> [VTQD_ComboKeyEn_flg]
  [VTQD_ComboKey1_enum] -> VTQD_ComboKey1_enum/1
  [VTQD_Function1Off1Pass_flg] -> VTQD_Key1Pass_flg/1
  [VTQD_ComboKey1_enum] -> Delay1/1
  Delay1/1 -> Maintain/1(Input)
  Data Type Conversion/1 -> [VTQD_ComboKey1_enum]  "VTQD_Function1Off1_enum"

== system tqd/TQD/Input_Convert/Input Signal Convert/Big Mike Combo V2 /Combo Key Detection/Function1 Alcohol Lock/Key2 ==
  VTQD_Function1CMD_enum : Inport
  VTQD_ComboKeyEn_flg : Inport  Port=2
  VTQD_ComboKeyReset_flg : Inport  Port=3
  VTQD_ComboKey1_enum : Inport  Port=4
  AND : Logic  Inputs=4  AllPortsSameDT=off  OutDataTypeStr=boolean
  Constant1 : Constant  Value=KTQD_Function1Off2_enum
  Constant2 : Constant  Value=ENUM_COMBOKEY_NONE
  Constant3 : Constant  Value=ENUM_COMBOKEY_NONE
  Constant4 : Constant  Value=ENUM_COMBOKEY_NONE  OutDataTypeStr=uint8
  Data Type Conversion : DataTypeConversion  OutDataTypeStr=uint8
  Delay : Delay  DelayLength=1  InitialCondition=uint8(0)
      settings: AttributesFormatString=%<InitialCondition>
  Delay1 : Delay  DelayLength=1  InitialCondition=uint8(0)
      settings: AttributesFormatString=%<InitialCondition>
  Delay2 : Delay  DelayLength=1  InitialCondition=uint8(0)
      settings: AttributesFormatString=%<InitialCondition>
  Detect Change : simulink/Logic and Bit Operations/Detect Change  vinit=boolean(0)  OutDataTypeStr=boolean
  Detect Increase : simulink/Logic and Bit Operations/Detect Increase  vinit=boolean(0)  OutDataTypeStr=boolean
  Equal : RelationalOperator  Operator===  OutDataTypeStr=boolean  RndMeth=Simplest
  Equal1 : RelationalOperator  Operator=~=  OutDataTypeStr=boolean  RndMeth=Simplest
  Equal2 : RelationalOperator  Operator=~=  OutDataTypeStr=boolean  RndMeth=Simplest
  Equal3 : RelationalOperator  Operator===  OutDataTypeStr=boolean  RndMeth=Simplest
  If : If  NumInputs=2  IfExpression=u1 ~=0  ElseIfExpressions=u2 ~= 0
  Maintain : Subsystem  TreatAsAtomicUnit=on
  Merge : Merge  Inputs=3
  OR : Logic  Operator=OR  AllPortsSameDT=off  OutDataTypeStr=boolean
  Reset : Subsystem  TreatAsAtomicUnit=on
  Write : Subsystem  TreatAsAtomicUnit=on
  VTQD_ComboKey2_enum : Outport
  VTQD_Key2Pass_flg : Outport  Port=2
  wires:
  [VTQD_Key2Pass_flg] -> VTQD_Key2Pass_flg/1
  [VTQD_ComboKey2_enum] -> VTQD_ComboKey2_enum/1
  VTQD_ComboKeyEn_flg/1 -> [VTQD_ComboKeyEn_flg]
  VTQD_ComboKeyReset_flg/1 -> [VTQD_ComboKeyReset_flg]
  VTQD_Function1CMD_enum/1 -> [VTQD_ComboKeyCMD_enum]
  Equal/1 -> [VTQD_Key2Pass_flg]  "VTQD_Function1Off2Pass_flg"
  Constant1/1 -> Equal/2
  [VTQD_ComboKey2_enum] -> Equal/1
  If/2 -> Write/Action
  Write/1(WriteCMD) -> Merge/2
  If/1 -> Reset/Action
  Detect Increase/1 -> OR/1
  AND/1 -> [VTQD_WriteComboCMD_flg]  "VTQD_WriteComboCMD_flg"
  [VTQD_ComboKeyCMD_enum] -> Write/1(Input)
  [VTQD_ComboKeyCMD_enum] -> Detect Change/1
  [VTQD_ResetComboKey_flg] -> If/1
  [VTQD_ComboKeyEn_flg] -> Detect Increase/1
  Detect Change/1 -> AND/1
  Maintain/1(KeepKey2) -> Merge/3
  Constant4/1 -> Equal1/2
  If/3 -> Maintain/Action
  Delay/1 -> Equal2/1
  Merge/1 -> Data Type Conversion/1
  Reset/1(ResetToZero) -> Merge/1
  Equal2/1 -> AND/3
  Constant2/1 -> Equal2/2
  Equal1/1 -> AND/2
  [VTQD_ComboKey1_enum] -> Delay/1
  [VTQD_ComboKeyReset_flg] -> OR/2
  [VTQD_ComboKeyCMD_enum] -> Equal1/1
  [VTQD_WriteComboCMD_flg] -> If/2
  OR/1 -> [VTQD_ResetComboKey_flg]  "VTQD_ResetComboKey_flg"
  VTQD_ComboKey1_enum/1 -> [VTQD_ComboKey1_enum]
  [VTQD_ComboKey2_enum] -> Delay1/1
  Constant3/1 -> Equal3/2
  Delay1/1 -> Equal3/1
  Equal3/1 -> AND/4
  Delay2/1 -> Maintain/1(Input)
  [VTQD_ComboKey2_enum] -> Delay2/1
  Data Type Conversion/1 -> [VTQD_ComboKey2_enum]  "VTQD_Function1Off2_enum"

== system tqd/TQD/Input_Convert/Input Signal Convert/Big Mike Combo V2 /Combo Key Detection/Function1 Alcohol Lock/Key3 ==
  VTQD_ComboKeyCMD_enum : Inport
  VTQD_ComboKeyEn_flg : Inport  Port=2
  VTQD_ComboKeyReset_flg : Inport  Port=3
  VTQD_ComboKey2_enum : Inport  Port=4
  AND : Logic  Inputs=4  AllPortsSameDT=off  OutDataTypeStr=boolean
  Constant1 : Constant  Value=KTQD_Function1Off3_enum
  Constant2 : Constant  Value=ENUM_COMBOKEY_NONE
  Constant3 : Constant  Value=ENUM_COMBOKEY_NONE
  Constant4 : Constant  Value=ENUM_COMBOKEY_NONE
  Data Type Conversion : DataTypeConversion  OutDataTypeStr=uint8
  Delay : Delay  DelayLength=1  InitialCondition=uint8(0)
      settings: AttributesFormatString=%<InitialCondition>
  Delay1 : Delay  DelayLength=1  InitialCondition=uint8(0)
      settings: AttributesFormatString=%<InitialCondition>
  Delay2 : Delay  DelayLength=1  InitialCondition=uint8(0)
      settings: AttributesFormatString=%<InitialCondition>
  Detect Change : simulink/Logic and Bit Operations/Detect Change  vinit=boolean(0)  OutDataTypeStr=boolean
  Detect Increase : simulink/Logic and Bit Operations/Detect Increase  vinit=boolean(0)  OutDataTypeStr=boolean
  Equal : RelationalOperator  Operator===  OutDataTypeStr=boolean  RndMeth=Simplest
  Equal1 : RelationalOperator  Operator=~=  OutDataTypeStr=boolean  RndMeth=Simplest
  Equal2 : RelationalOperator  Operator=~=  OutDataTypeStr=boolean  RndMeth=Simplest
  Equal3 : RelationalOperator  Operator===  OutDataTypeStr=boolean  RndMeth=Simplest
  If : If  NumInputs=2  IfExpression=u1 ~=0  ElseIfExpressions=u2 ~= 0
  Maintain : Subsystem  TreatAsAtomicUnit=on
  Merge : Merge  Inputs=3
  OR : Logic  Operator=OR  AllPortsSameDT=off  OutDataTypeStr=boolean
  Reset : Subsystem  TreatAsAtomicUnit=on
  Write : Subsystem  TreatAsAtomicUnit=on
  VTQD_ComboKey3_enum : Outport
  VTQD_Key3Pass_flg : Outport  Port=2
  wires:
  VTQD_ComboKey2_enum/1 -> [VTQD_ComboKey2_enum]
  OR/1 -> [VTQD_ResetComboKey_flg]  "VTQD_ResetComboKey_flg"
  [VTQD_WriteComboCMD_flg] -> If/2
  [VTQD_ComboKeyCMD_enum] -> Equal1/1
  [VTQD_ComboKeyReset_flg] -> OR/2
  [VTQD_ComboKey2_enum] -> Delay/1
  Equal1/1 -> AND/2
  Constant2/1 -> Equal2/2
  Equal2/1 -> AND/3
  Reset/1(ResetToZero) -> Merge/1
  Merge/1 -> Data Type Conversion/1
  Delay/1 -> Equal2/1
  If/3 -> Maintain/Action
  Constant4/1 -> Equal1/2
  Maintain/1(KeepKey3) -> Merge/3
  Detect Change/1 -> AND/1
  [VTQD_ComboKeyEn_flg] -> Detect Increase/1
  [VTQD_ResetComboKey_flg] -> If/1
  [VTQD_ComboKeyCMD_enum] -> Detect Change/1
  [VTQD_ComboKeyCMD_enum] -> Write/1(Input)
  AND/1 -> [VTQD_WriteComboCMD_flg]  "VTQD_WriteComboCMD_flg"
  Detect Increase/1 -> OR/1
  If/1 -> Reset/Action
  Write/1(WriteCMD) -> Merge/2
  If/2 -> Write/Action
  Constant1/1 -> Equal/2
  Equal/1 -> [VTQD_Function1Off3Pass_flg]  "VTQD_Function1Off3Pass_flg"
  VTQD_ComboKeyCMD_enum/1 -> [VTQD_ComboKeyCMD_enum]
  VTQD_ComboKeyReset_flg/1 -> [VTQD_ComboKeyReset_flg]
  VTQD_ComboKeyEn_flg/1 -> [VTQD_ComboKeyEn_flg]
  [VTQD_ComboKey3_enum] -> VTQD_ComboKey3_enum/1
  [VTQD_ComboKey3_enum] -> Equal/1
  [VTQD_Function1Off3Pass_flg] -> VTQD_Key3Pass_flg/1
  Delay1/1 -> Equal3/1
  Equal3/1 -> AND/4
  Constant3/1 -> Equal3/2
  [VTQD_ComboKey3_enum] -> Delay1/1
  Delay2/1 -> Maintain/1(Input)
  [VTQD_ComboKey3_enum] -> Delay2/1
  Data Type Conversion/1 -> [VTQD_ComboKey3_enum]  "VTQD_Function1Off3_enum"

== system tqd/TQD/Input_Convert/Input Signal Convert/Big Mike Combo V2 /Combo Key Detection/Function1 Alcohol Lock/Key4 ==
  VTQD_ComboKeyCMD_enum : Inport
  VTQD_ComboKeyEn_flg : Inport  Port=2
  VTQD_ComboKeyReset_flg : Inport  Port=3
  VTQD_ComboKey3_enum : Inport  Port=4
  AND : Logic  Inputs=4  AllPortsSameDT=off  OutDataTypeStr=boolean
  Constant1 : Constant  Value=KTQD_Function1Off4_enum
  Constant2 : Constant  Value=ENUM_COMBOKEY_NONE
  Constant3 : Constant  Value=ENUM_COMBOKEY_NONE
  Constant4 : Constant  Value=ENUM_COMBOKEY_NONE
  Data Type Conversion : DataTypeConversion  OutDataTypeStr=uint8
  Delay : Delay  DelayLength=1  InitialCondition=uint8(0)
      settings: AttributesFormatString=%<InitialCondition>
  Delay1 : Delay  DelayLength=1  InitialCondition=uint8(0)
      settings: AttributesFormatString=%<InitialCondition>
  Delay2 : Delay  DelayLength=1  InitialCondition=uint8(0)
      settings: AttributesFormatString=%<InitialCondition>
  Detect Change : simulink/Logic and Bit Operations/Detect Change  vinit=boolean(0)  OutDataTypeStr=boolean
  Detect Increase : simulink/Logic and Bit Operations/Detect Increase  vinit=boolean(0)  OutDataTypeStr=boolean
  Equal : RelationalOperator  Operator===  OutDataTypeStr=boolean  RndMeth=Simplest
  Equal1 : RelationalOperator  Operator=~=  OutDataTypeStr=boolean  RndMeth=Simplest
  Equal2 : RelationalOperator  Operator=~=  OutDataTypeStr=boolean  RndMeth=Simplest
  Equal3 : RelationalOperator  Operator===  OutDataTypeStr=boolean  RndMeth=Simplest
  If : If  NumInputs=2  IfExpression=u1 ~=0  ElseIfExpressions=u2 ~= 0
  Maintain : Subsystem  TreatAsAtomicUnit=on
  Merge : Merge  Inputs=3
  OR : Logic  Operator=OR  AllPortsSameDT=off  OutDataTypeStr=boolean
  Reset : Subsystem  TreatAsAtomicUnit=on
  Write : Subsystem  TreatAsAtomicUnit=on
  VTQD_ComboKey4_enum : Outport
  VTQD_Key4Pass_flg : Outport  Port=2
  wires:
  [VTQD_ComboKey4_enum] -> Equal/1
  VTQD_ComboKeyEn_flg/1 -> [VTQD_ComboKeyEn_flg]
  VTQD_ComboKeyReset_flg/1 -> [VTQD_ComboKeyReset_flg]
  VTQD_ComboKeyCMD_enum/1 -> [VTQD_ComboKeyCMD_enum]
  Equal/1 -> [VTQD_Function1Off4Pass_flg]  "VTQD_Function1Off4Pass_flg"
  Constant1/1 -> Equal/2
  If/2 -> Write/Action
  Write/1(WriteCMD) -> Merge/2
  If/1 -> Reset/Action
  Detect Increase/1 -> OR/1
  AND/1 -> [VTQD_WriteComboCMD_flg]  "VTQD_WriteComboCMD_flg"
  [VTQD_ComboKeyCMD_enum] -> Write/1(Input)
  [VTQD_ComboKeyCMD_enum] -> Detect Change/1
  [VTQD_ResetComboKey_flg] -> If/1
  [VTQD_ComboKeyEn_flg] -> Detect Increase/1
  Detect Change/1 -> AND/1
  Maintain/1(KeepKey4) -> Merge/3
  Constant4/1 -> Equal1/2
  If/3 -> Maintain/Action
  Delay/1 -> Equal2/1
  Merge/1 -> Data Type Conversion/1
  Reset/1(ResetToZero) -> Merge/1
  Equal2/1 -> AND/3
  Constant2/1 -> Equal2/2
  Equal1/1 -> AND/2
  [VTQD_ComboKey3_enum] -> Delay/1
  [VTQD_ComboKeyReset_flg] -> OR/2
  [VTQD_ComboKeyCMD_enum] -> Equal1/1
  [VTQD_WriteComboCMD_flg] -> If/2
  OR/1 -> [VTQD_ResetComboKey_flg]  "VTQD_ResetComboKey_flg"
  VTQD_ComboKey3_enum/1 -> [VTQD_ComboKey3_enum]
  [VTQD_ComboKey4_enum] -> Delay1/1
  Constant3/1 -> Equal3/2
  Delay1/1 -> Equal3/1
  Equal3/1 -> AND/4
  [VTQD_Function1Off4Pass_flg] -> VTQD_Key4Pass_flg/1
  [VTQD_ComboKey4_enum] -> VTQD_ComboKey4_enum/1
  [VTQD_ComboKey4_enum] -> Delay2/1
  Delay2/1 -> Maintain/1(Input)
  Data Type Conversion/1 -> [VTQD_ComboKey4_enum]  "VTQD_Function1Off4_enum"

== system tqd/TQD/Input_Convert/Input Signal Convert/Big Mike Combo V2 /Combo Key Detection/Function1 Alcohol Lock/Key5 ==
  VTQD_ComboKeyCMD_enum : Inport
  VTQD_ComboKeyEn_flg : Inport  Port=2
  VTQD_ComboKeyReset_flg : Inport  Port=3
  VTQD_ComboKey4_enum : Inport  Port=4
  AND : Logic  Inputs=4  AllPortsSameDT=off  OutDataTypeStr=boolean
  Constant1 : Constant  Value=KTQD_Function1Off5_enum
  Constant2 : Constant  Value=ENUM_COMBOKEY_NONE
  Constant3 : Constant  Value=ENUM_COMBOKEY_NONE
  Constant4 : Constant  Value=ENUM_COMBOKEY_NONE
  Data Type Conversion : DataTypeConversion  OutDataTypeStr=uint8
  Delay : Delay  DelayLength=1  InitialCondition=uint8(0)
      settings: AttributesFormatString=%<InitialCondition>
  Delay1 : Delay  DelayLength=1  InitialCondition=uint8(0)
      settings: AttributesFormatString=%<InitialCondition>
  Delay2 : Delay  DelayLength=1  InitialCondition=uint8(0)
      settings: AttributesFormatString=%<InitialCondition>
  Detect Change : simulink/Logic and Bit Operations/Detect Change  vinit=boolean(0)  OutDataTypeStr=boolean
  Detect Increase : simulink/Logic and Bit Operations/Detect Increase  vinit=boolean(0)  OutDataTypeStr=boolean
  Equal : RelationalOperator  Operator===  OutDataTypeStr=boolean  RndMeth=Simplest
  Equal1 : RelationalOperator  Operator=~=  OutDataTypeStr=boolean  RndMeth=Simplest
  Equal2 : RelationalOperator  Operator=~=  OutDataTypeStr=boolean  RndMeth=Simplest
  Equal3 : RelationalOperator  Operator===  OutDataTypeStr=boolean  RndMeth=Simplest
  If : If  NumInputs=2  IfExpression=u1 ~=0  ElseIfExpressions=u2 ~= 0
  Maintain : Subsystem  TreatAsAtomicUnit=on
  Merge : Merge  Inputs=3
  OR : Logic  Operator=OR  AllPortsSameDT=off  OutDataTypeStr=boolean
  Reset : Subsystem  TreatAsAtomicUnit=on
  Write : Subsystem  TreatAsAtomicUnit=on
  VTQD_ComboKey5_enum : Outport
  VTQD_Key5Pass_flg : Outport  Port=2
  wires:
  [VTQD_Key5Pass_flg] -> VTQD_Key5Pass_flg/1
  Equal3/1 -> AND/4
  Delay1/1 -> Equal3/1
  Constant3/1 -> Equal3/2
  [VTQD_ComboKey5_enum] -> Delay1/1
  VTQD_ComboKey4_enum/1 -> [VTQD_ComboKey4_enum]
  OR/1 -> [VTQD_ResetComboKey_flg]  "VTQD_ResetComboKey_flg"
  [VTQD_WriteComboCMD_flg] -> If/2
  [VTQD_ComboKeyCMD_enum] -> Equal1/1
  [VTQD_ComboKeyReset_flg] -> OR/2
  [VTQD_ComboKey4_enum] -> Delay/1
  Equal1/1 -> AND/2
  Constant2/1 -> Equal2/2
  Equal2/1 -> AND/3
  Reset/1(ResetToZero) -> Merge/1
  Merge/1 -> Data Type Conversion/1
  Delay/1 -> Equal2/1
  If/3 -> Maintain/Action
  Constant4/1 -> Equal1/2
  Maintain/1(KeepKey5) -> Merge/3
  Detect Change/1 -> AND/1
  [VTQD_ComboKeyEn_flg] -> Detect Increase/1
  [VTQD_ResetComboKey_flg] -> If/1
  [VTQD_ComboKeyCMD_enum] -> Detect Change/1
  [VTQD_ComboKeyCMD_enum] -> Write/1(Input)
  AND/1 -> [VTQD_WriteComboCMD_flg]  "VTQD_WriteComboCMD_flg"
  Detect Increase/1 -> OR/1
  If/1 -> Reset/Action
  Write/1(WriteCMD) -> Merge/2
  If/2 -> Write/Action
  Constant1/1 -> Equal/2
  Equal/1 -> [VTQD_Key5Pass_flg]  "VTQD_Function1Off5Pass_flg"
  VTQD_ComboKeyCMD_enum/1 -> [VTQD_ComboKeyCMD_enum]
  VTQD_ComboKeyReset_flg/1 -> [VTQD_ComboKeyReset_flg]
  VTQD_ComboKeyEn_flg/1 -> [VTQD_ComboKeyEn_flg]
  [VTQD_ComboKey5_enum] -> Equal/1
  [VTQD_ComboKey5_enum] -> VTQD_ComboKey5_enum/1
  [VTQD_ComboKey5_enum] -> Delay2/1
  Delay2/1 -> Maintain/1(Input)
  Data Type Conversion/1 -> [VTQD_ComboKey5_enum]  "VTQD_Function1Off5_enum"

== system tqd/TQD/Input_Convert/Input Signal Convert/Big Mike Combo V2 /Combo Key Detection/Function1 Alcohol Lock/Key6 ==
  VTQD_ComboKeyCMD_enum : Inport
  VTQD_ComboKeyEn_flg : Inport  Port=2
  VTQD_ComboKeyReset_flg : Inport  Port=3
  VTQD_ComboKey5_enum : Inport  Port=4
  AND : Logic  Inputs=4  AllPortsSameDT=off  OutDataTypeStr=boolean
  Constant1 : Constant  Value=KTQD_Function1Off6_enum
  Constant2 : Constant  Value=ENUM_COMBOKEY_NONE
  Constant3 : Constant  Value=ENUM_COMBOKEY_NONE
  Constant4 : Constant  Value=ENUM_COMBOKEY_NONE
  Data Type Conversion : DataTypeConversion  OutDataTypeStr=uint8
  Delay : Delay  DelayLength=1  InitialCondition=uint8(0)
      settings: AttributesFormatString=%<InitialCondition>
  Delay1 : Delay  Description=%<InitialCondition>  DelayLength=1  InitialCondition=uint8(0)
  Delay2 : Delay  DelayLength=1  InitialCondition=uint8(0)
      settings: AttributesFormatString=%<InitialCondition>
  Detect Change : simulink/Logic and Bit Operations/Detect Change  vinit=boolean(0)  OutDataTypeStr=boolean
  Detect Increase : simulink/Logic and Bit Operations/Detect Increase  vinit=boolean(0)  OutDataTypeStr=boolean
  Equal : RelationalOperator  Operator===  OutDataTypeStr=boolean  RndMeth=Simplest
  Equal1 : RelationalOperator  Operator=~=  OutDataTypeStr=boolean  RndMeth=Simplest
  Equal2 : RelationalOperator  Operator=~=  OutDataTypeStr=boolean  RndMeth=Simplest
  Equal3 : RelationalOperator  Operator===  OutDataTypeStr=boolean  RndMeth=Simplest
  If : If  NumInputs=2  IfExpression=u1 ~=0  ElseIfExpressions=u2 ~= 0
  Maintain : Subsystem  TreatAsAtomicUnit=on
  Merge : Merge  Inputs=3
  OR : Logic  Operator=OR  AllPortsSameDT=off  OutDataTypeStr=boolean
  Reset : Subsystem  TreatAsAtomicUnit=on
  Write : Subsystem  TreatAsAtomicUnit=on
  VTQD_ComboKey6_enum : Outport
  VTQD_Key6Pass_flg : Outport  Port=2
  wires:
  [VTQD_ComboKey6_enum] -> VTQD_ComboKey6_enum/1
  [VTQD_ComboKey6_enum] -> Equal/1
  VTQD_ComboKeyEn_flg/1 -> [VTQD_ComboKeyEn_flg]
  VTQD_ComboKeyReset_flg/1 -> [VTQD_ComboKeyReset_flg]
  VTQD_ComboKeyCMD_enum/1 -> [VTQD_ComboKeyCMD_enum]
  Equal/1 -> [VTQD_Key6Pass_flg]  "VTQD_Function1Off6Pass_flg"
  Constant1/1 -> Equal/2
  If/2 -> Write/Action
  Write/1(WriteCMD) -> Merge/2
  If/1 -> Reset/Action
  Detect Increase/1 -> OR/1
  AND/1 -> [VTQD_WriteComboCMD_flg]  "VTQD_WriteComboCMD_flg"
  [VTQD_ComboKeyCMD_enum] -> Write/1(Input)
  [VTQD_ComboKeyCMD_enum] -> Detect Change/1
  [VTQD_ResetComboKey_flg] -> If/1
  [VTQD_ComboKeyEn_flg] -> Detect Increase/1
  Detect Change/1 -> AND/1
  Maintain/1(KeepKey6) -> Merge/3
  Constant4/1 -> Equal1/2
  If/3 -> Maintain/Action
  Delay/1 -> Equal2/1
  Merge/1 -> Data Type Conversion/1
  Reset/1(ResetToZero) -> Merge/1
  Equal2/1 -> AND/3
  Constant2/1 -> Equal2/2
  Equal1/1 -> AND/2
  [VTQD_ComboKey5_enum] -> Delay/1
  [VTQD_ComboKeyReset_flg] -> OR/2
  [VTQD_ComboKeyCMD_enum] -> Equal1/1
  [VTQD_WriteComboCMD_flg] -> If/2
  OR/1 -> [VTQD_ResetComboKey_flg]  "VTQD_ResetComboKey_flg"
  VTQD_ComboKey5_enum/1 -> [VTQD_ComboKey5_enum]
  [VTQD_ComboKey6_enum] -> Delay1/1
  Constant3/1 -> Equal3/2
  Delay1/1 -> Equal3/1
  Equal3/1 -> AND/4
  [VTQD_Key6Pass_flg] -> VTQD_Key6Pass_flg/1
  Delay2/1 -> Maintain/1(Input)
  [VTQD_ComboKey6_enum] -> Delay2/1
  Data Type Conversion/1 -> [VTQD_ComboKey6_enum]  "VTQD_Function1Off6_enum"

== system tqd/TQD/Input_Convert/Input Signal Convert/Big Mike Combo V2 /Combo Key Detection/Function1 Alcohol Lock/Key7 ==
  VTQD_ComboKeyCMD_enum : Inport
  VTQD_ComboKeyEn_flg : Inport  Port=2
  VTQD_ComboKeyReset_flg : Inport  Port=3
  VTQD_ComboKey6_enum : Inport  Port=4
  AND : Logic  Inputs=4  AllPortsSameDT=off  OutDataTypeStr=boolean
  Constant1 : Constant  Value=KTQD_Function1Off7_enum
  Constant2 : Constant  Value=ENUM_COMBOKEY_NONE  OutDataTypeStr=uint8
  Constant3 : Constant  Value=ENUM_COMBOKEY_NONE
  Constant4 : Constant  Value=ENUM_COMBOKEY_NONE  OutDataTypeStr=uint8
  Data Type Conversion : DataTypeConversion  OutDataTypeStr=uint8
  Delay : Delay  DelayLength=1  InitialCondition=uint8(0)
      settings: AttributesFormatString=%<InitialCondition>
  Delay1 : Delay  DelayLength=1  InitialCondition=uint8(0)
      settings: AttributesFormatString=%<InitialCondition>
  Delay2 : Delay  DelayLength=1  InitialCondition=uint8(0)
      settings: AttributesFormatString=%<InitialCondition>
  Detect Change : simulink/Logic and Bit Operations/Detect Change  vinit=boolean(0)  OutDataTypeStr=boolean
  Detect Increase : simulink/Logic and Bit Operations/Detect Increase  vinit=boolean(0)  OutDataTypeStr=boolean
  Equal : RelationalOperator  Operator===  OutDataTypeStr=boolean  RndMeth=Simplest
  Equal1 : RelationalOperator  Operator=~=  OutDataTypeStr=boolean  RndMeth=Simplest
  Equal2 : RelationalOperator  Operator=~=  OutDataTypeStr=boolean  RndMeth=Simplest
  Equal3 : RelationalOperator  Operator===  OutDataTypeStr=boolean  RndMeth=Simplest
  If : If  NumInputs=2  IfExpression=u1 ~=0  ElseIfExpressions=u2 ~= 0
  Maintain : Subsystem  TreatAsAtomicUnit=on
  Merge : Merge  Inputs=3
  OR : Logic  Operator=OR  AllPortsSameDT=off  OutDataTypeStr=boolean
  Reset : Subsystem  TreatAsAtomicUnit=on
  Write : Subsystem  TreatAsAtomicUnit=on
  VTQD_ComboKey7_enum : Outport
  VTQD_Key7Pass_flg : Outport  Port=2
  wires:
  [VTQD_Key7Pass_flg] -> VTQD_Key7Pass_flg/1
  Equal3/1 -> AND/4
  Delay1/1 -> Equal3/1
  Constant3/1 -> Equal3/2
  [VTQD_ComboKey7_enum] -> Delay1/1
  VTQD_ComboKey6_enum/1 -> [VTQD_ComboKey6_enum]
  OR/1 -> [VTQD_ResetComboKey_flg]  "VTQD_ResetComboKey_flg"
  [VTQD_WriteComboCMD_flg] -> If/2
  [VTQD_ComboKeyCMD_enum] -> Equal1/1
  [VTQD_ComboKeyReset_flg] -> OR/2
  [VTQD_ComboKey6_enum] -> Delay/1
  Equal1/1 -> AND/2
  Constant2/1 -> Equal2/2
  Equal2/1 -> AND/3
  Reset/1(ResetToZero) -> Merge/1
  Merge/1 -> Data Type Conversion/1
  Delay/1 -> Equal2/1
  If/3 -> Maintain/Action
  Constant4/1 -> Equal1/2
  Maintain/1(KeepKey7) -> Merge/3
  Detect Change/1 -> AND/1
  [VTQD_ComboKeyEn_flg] -> Detect Increase/1
  [VTQD_ResetComboKey_flg] -> If/1
  [VTQD_ComboKeyCMD_enum] -> Detect Change/1
  [VTQD_ComboKeyCMD_enum] -> Write/1(Input)
  AND/1 -> [VTQD_WriteComboCMD_flg]  "VTQD_WriteComboCMD_flg"
  Detect Increase/1 -> OR/1
  If/1 -> Reset/Action
  Write/1(WriteCMD) -> Merge/2
  If/2 -> Write/Action
  Constant1/1 -> Equal/2
  Equal/1 -> [VTQD_Key7Pass_flg]  "VTQD_Function1Off7Pass_flg"
  VTQD_ComboKeyCMD_enum/1 -> [VTQD_ComboKeyCMD_enum]
  VTQD_ComboKeyReset_flg/1 -> [VTQD_ComboKeyReset_flg]
  VTQD_ComboKeyEn_flg/1 -> [VTQD_ComboKeyEn_flg]
  [VTQD_ComboKey7_enum] -> Equal/1
  [VTQD_ComboKey7_enum] -> VTQD_ComboKey7_enum/1
  [VTQD_ComboKey7_enum] -> Delay2/1
  Delay2/1 -> Maintain/1(Input)
  Data Type Conversion/1 -> [VTQD_ComboKey7_enum]  "VTQD_Function1Off7_enum"
